simulink model "Citation_FlightGear_v2"  (R2026a)
settings: Solver=ode5  StopTime=10  FixedStep=0.01  EnableMultiTasking=on
InitFcn:
  | run('initcit.m')
  | run('id_init.m')
values from neighbouring files (symbols this model uses):
  beta_ref_max = 5*pi/180    (= 0.0872664625997)    [id_init.m]
  K_beta = 2    [id_init.m]
  K_da_to_p = p_ref_max/0.65    (= 0.537024385229)    [id_init.m]
  K_de_to_q = q_ref_max/0.35    (= 0.49866550057)    [id_init.m]
  K_dr_to_beta = beta_ref_max/0.38    (= 0.229648585789)    [id_init.m]
  Kaw_p = 1/Taw_p    (= 2)    [id_init.m]
  Kaw_q = 1/Taw_q    (= 2)    [id_init.m]
  Kaw_r = 1/Taw_r    (= 2)    [id_init.m]
  Ki_p = 5.0    (= 5)    [id_init.m]
  Ki_p_classical = -0.5    [id_init.m]
  Ki_q = 5.0    (= 5)    [id_init.m]
  Ki_q_classical = -0.1    [id_init.m]
  Ki_r = 5.0    (= 5)    [id_init.m]
  Ki_r_classical = -0.1    [id_init.m]
  Kp_p = 4.5    [id_init.m]
  Kp_p_classical = -1    [id_init.m]
  Kp_q = 4.5    [id_init.m]
  Kp_q_classical = -2    [id_init.m]
  Kp_r = 4.5    [id_init.m]
  Kp_r_classical = -2    [id_init.m]
  p_ref_max = 20*pi/180    (= 0.349065850399)    [id_init.m]
  PL0 = 10000*eye(6)    [id_init.m]
  PM0 = 10000*eye(4)    [id_init.m]
  PN0 = 10000*eye(6)    [id_init.m]
  PX0 = 10000*eye(5)    [id_init.m]
  PY0 = 10000*eye(6)    [id_init.m]
  PZ0 = 10000*eye(4)    [id_init.m]
  q_ref_max = 10*pi/180    (= 0.174532925199)    [id_init.m]
  r_ref_max = 10*pi/180    (= 0.174532925199)    [id_init.m]
  tau_cmd = 0.5    [id_init.m]
  thetaL0 = [       7.0957952465296537e-06 ... (first row only)    [id_init.m]
  thetaM0 = [       1.2280209971618383e-02 ... (first row only)    [id_init.m]
  thetaN0 = [      -4.9609095125384690e-06 ... (first row only)    [id_init.m]
  thetaX0 = zeros(5,1)    [id_init.m]
  thetaY0 = zeros(6,1)    [id_init.m]
  thetaZ0 = zeros(4,1)    [id_init.m]
  TL = 7.0875e-06    [id_init.m]
  TM = 3.2564e-06    [id_init.m]
  TN = 5.4692e-07    [id_init.m]
  TX = 2.2784e-06    [id_init.m]
  TY = 8.0633e-07    [id_init.m]
  TZ = 2.8004e-05    [id_init.m]
  Vw915 = 0    [initcit.m]
  winddir = -27*(pi/180)    (= -0.471238898038)    [initcit.m]
  x0 = []    [cessnac550_3d_sfnc.m]
undefined symbols (not defined in the file or in its folder): chord, cv1, cv2, cv3, cv4, deltagmax1, deltagmax2, deltagmax3, deltagmax4, Deng, ealphag, ealphas, g0, hDME, hGS, kt1, kt2, kt3, lh, massinit, matbuaf, matdaf, matdam, matdbbf, matdeaf, matdgaf, matdqaf, matduaf, matdwaw, matedhr, mateif, matelhr, matemhr, matemv1, matemv2, matemve, matetam, mateuaf, matfaaf, matfaxl, matff, matibaf, matibb, matibmh, matipaf, matipmh, matiraf, matiuaf, matiwaf, matlaf, matlam, matleaf, matleam, matlgaf, matlqaf, matluaf, matmaaf, matmaam, matmaf, matmam ... (+78)
libraries: simulink x13, aerolibfltsims x3, aerolibconvert2 x2, aerolibobsolete x1, aerolibanimutils x1
(part 5 of 5)

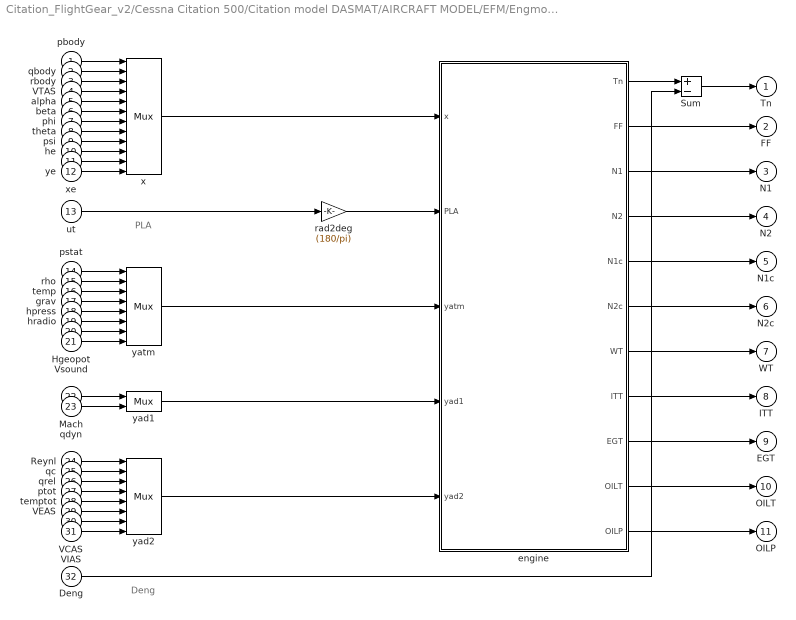
== system Citation_FlightGear_v2/Cessna Citation 500/Citation model DASMAT/AIRCRAFT MODEL/EFM/Engmod/Citation eng_mod/Subsystem1/JT15 Dynamic1/Subsystem ==
  note: Deng
  note: PLA
  pbody : Inport
  qbody : Inport  Port=2
  rbody : Inport  Port=3
  VTAS : Inport  Port=4
  alpha : Inport  Port=5
  beta : Inport  Port=6
  phi : Inport  Port=7
  theta : Inport  Port=8
  psi : Inport  Port=9
  he : Inport  Port=10
  xe : Inport  Port=11
  ye : Inport  Port=12
  ut : Inport  Port=13
  pstat : Inport  Port=14
  rho : Inport  Port=15
  temp : Inport  Port=16
  grav : Inport  Port=17
  hpress : Inport  Port=18
  hradio : Inport  Port=19
  Hgeopot : Inport  Port=20
  Vsound : Inport  Port=21
  Mach : Inport  Port=22
  qdyn : Inport  Port=23
  Reynl : Inport  Port=24
  qc : Inport  Port=25
  qrel : Inport  Port=26
  ptot : Inport  Port=27
  temptot : Inport  Port=28
  VEAS : Inport  Port=29
  VCAS : Inport  Port=30
  VIAS : Inport  Port=31
  Deng : Inport  Port=32
  Sum : Sum  Inputs=+-  InputSameDT=on  SaturateOnIntegerOverflow=on  OutDataTypeStr=Inherit: Same as first input
  engine : Subsystem
  rad2deg : Gain  Gain=(180/pi)  SaturateOnIntegerOverflow=on  OutDataTypeStr=Inherit: Same as input  ParamDataTypeStr=Inherit: Same as input
  x : Mux  Inputs=12
  yad1 : Mux  Inputs=2
  yad2 : Mux  Inputs=8
  yatm : Mux  Inputs=8
  Tn : Outport
  FF : Outport  Port=2
  N1 : Outport  Port=3
  N2 : Outport  Port=4
  N1c : Outport  Port=5
  N2c : Outport  Port=6
  WT : Outport  Port=7
  ITT : Outport  Port=8
  EGT : Outport  Port=9
  OILT : Outport  Port=10
  OILP : Outport  Port=11
  wires:
  Deng/1 -> Sum/2
  engine/1(Tn) -> Sum/1
  Sum/1 -> Tn/1
  Vsound/1 -> yatm/8
  engine/11(OILP) -> OILP/1
  engine/10(OILT) -> OILT/1
  rad2deg/1 -> engine/2(PLA)
  ut/1 -> rad2deg/1
  engine/9(EGT) -> EGT/1
  engine/8(ITT) -> ITT/1
  engine/7(WT) -> WT/1
  engine/6(N2c) -> N2c/1
  engine/5(N1c) -> N1c/1
  engine/4(N2) -> N2/1
  engine/3(N1) -> N1/1
  engine/2(FF) -> FF/1
  yad1/1 -> engine/4(yad1)
  yatm/1 -> engine/3(yatm)
  yad2/1 -> engine/5(yad2)
  qdyn/1 -> yad1/2
  Mach/1 -> yad1/1
  Reynl/1 -> yad2/1
  qc/1 -> yad2/2
  VCAS/1 -> yad2/7
  temptot/1 -> yad2/5
  qrel/1 -> yad2/3
  VIAS/1 -> yad2/8
  VEAS/1 -> yad2/6
  ptot/1 -> yad2/4
  ye/1 -> x/12
  xe/1 -> x/11
  he/1 -> x/10
  psi/1 -> x/9
  VTAS/1 -> x/4
  beta/1 -> x/6
  theta/1 -> x/8
  rbody/1 -> x/3
  alpha/1 -> x/5
  phi/1 -> x/7
  qbody/1 -> x/2
  pbody/1 -> x/1
  pstat/1 -> yatm/1
  rho/1 -> yatm/2
  Hgeopot/1 -> yatm/7
  hpress/1 -> yatm/5
  temp/1 -> yatm/3
  hradio/1 -> yatm/6
  grav/1 -> yatm/4
  x/1 -> engine/1(x)

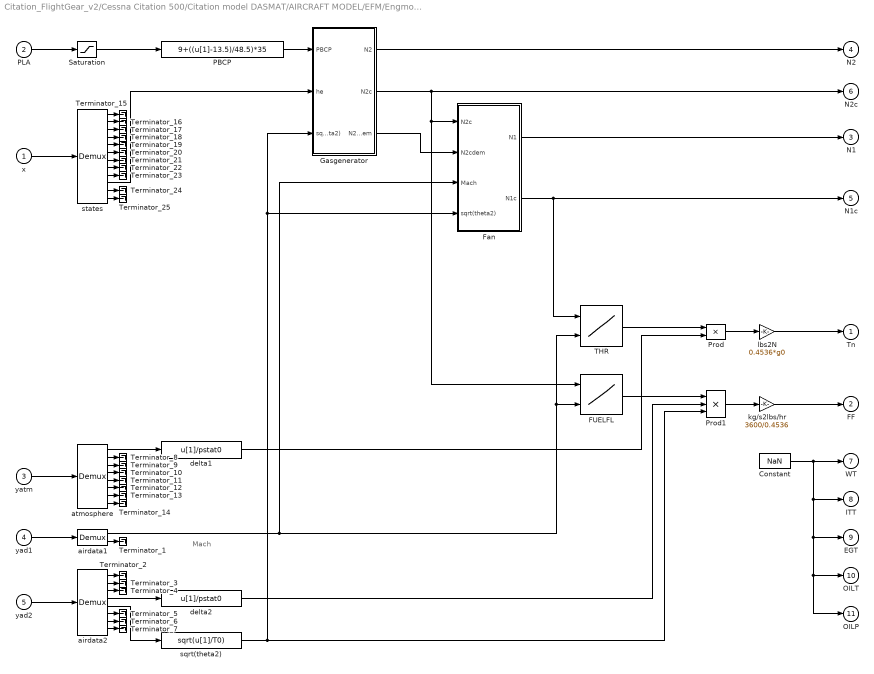
== system Citation_FlightGear_v2/Cessna Citation 500/Citation model DASMAT/AIRCRAFT MODEL/EFM/Engmod/Citation eng_mod/Subsystem1/JT15 Dynamic/Subsystem/engine ==
  note: Mach
  x : Inport
  PLA : Inport  Port=2
  yatm : Inport  Port=3
  yad1 : Inport  Port=4
  yad2 : Inport  Port=5
  Constant : Constant  Value=NaN
  FUELFL : Lookup2D  RowIndex=matff(2:14,1)  ColumnIndex=matff(1,2:14)  Table=matff(2:14,2:14)
  Fan : Subsystem
  Gasgenerator : Subsystem
  PBCP : Fcn  Expr=9+((u[1]-13.5)/48.5)*35
  Prod : Product  InputSameDT=on  SaturateOnIntegerOverflow=on  OutDataTypeStr=Inherit: Same as first input
  Prod1 : Product  Inputs=3  InputSameDT=on  SaturateOnIntegerOverflow=on  OutDataTypeStr=Inherit: Same as first input
  Saturation : Saturate  UpperLimit=62  LowerLimit=13.5
  THR : Lookup2D  RowIndex=matthr(2:12,1)  ColumnIndex=matthr(1,2:12)  Table=matthr(2:12,2:12)
  Terminator_{1..25} (25 alike) : Terminator
  airdata1 : Demux  Outputs=2
      settings: DisplayOption=none
  airdata2 : Demux  Outputs=8
      settings: DisplayOption=none
  atmosphere : Demux  Outputs=8
      settings: DisplayOption=none
  delta1 : Fcn  Expr=u[1]/pstat0
  delta2 : Fcn  Expr=u[1]/pstat0
  kg/s2lbs/hr : Gain  Gain=3600/0.4536  SaturateOnIntegerOverflow=on  OutDataTypeStr=Inherit: Same as input  ParamDataTypeStr=Inherit: Same as input
  lbs2N : Gain  Gain=0.4536*g0  SaturateOnIntegerOverflow=on  OutDataTypeStr=Inherit: Same as input  ParamDataTypeStr=Inherit: Same as input
  sqrt(theta2) : Fcn  Expr=sqrt(u[1]/T0)
  states : Demux  Outputs=12
      settings: DisplayOption=none
  Tn : Outport
  FF : Outport  Port=2
  N1 : Outport  Port=3
  N2 : Outport  Port=4
  N1c : Outport  Port=5
  N2c : Outport  Port=6
  WT : Outport  Port=7
  ITT : Outport  Port=8
  EGT : Outport  Port=9
  OILT : Outport  Port=10
  OILP : Outport  Port=11
  wires:
  states/12 -> Terminator_25/1
  states/11 -> Terminator_24/1
  states/9 -> Terminator_23/1
  states/8 -> Terminator_22/1
  states/7 -> Terminator_21/1
  states/6 -> Terminator_20/1
  states/5 -> Terminator_19/1
  states/4 -> Terminator_18/1
  states/3 -> Terminator_17/1
  states/2 -> Terminator_16/1
  states/1 -> Terminator_15/1
  atmosphere/8 -> Terminator_14/1
  atmosphere/7 -> Terminator_13/1
  atmosphere/6 -> Terminator_12/1
  atmosphere/5 -> Terminator_11/1
  atmosphere/4 -> Terminator_10/1
  atmosphere/3 -> Terminator_9/1
  atmosphere/2 -> Terminator_8/1
  airdata2/8 -> Terminator_7/1
  airdata2/7 -> Terminator_6/1
  airdata2/6 -> Terminator_5/1
  airdata2/3 -> Terminator_4/1
  airdata2/2 -> Terminator_3/1
  airdata2/1 -> Terminator_2/1
  airdata1/2 -> Terminator_1/1
  Fan/2(N1c) -> THR/1, N1c/1
  Gasgenerator/2(N2c) -> Fan/1(N2c), FUELFL/1, N2c/1
  Gasgenerator/3(N2cdem) -> Fan/2(N2cdem)
  airdata1/1 -> Fan/3(Mach), FUELFL/2, THR/2
  Fan/1(N1) -> N1/1
  sqrt(theta2)/1 -> Fan/4(sqrt(theta2)), Gasgenerator/3(sqrt(theta2)), Prod1/3
  yad2/1 -> airdata2/1
  yad1/1 -> airdata1/1
  yatm/1 -> atmosphere/1
  airdata2/4 -> delta2/1
  airdata2/5 -> sqrt(theta2)/1
  Constant/1 -> ITT/1, EGT/1, OILT/1, OILP/1, WT/1
  Gasgenerator/1(N2) -> N2/1
  delta1/1 -> Prod/2
  Prod/1 -> lbs2N/1
  THR/1 -> Prod/1
  lbs2N/1 -> Tn/1
  states/10 -> Gasgenerator/2(he)
  delta2/1 -> Prod1/2
  atmosphere/1 -> delta1/1
  Prod1/1 -> kg/s2lbs/hr/1
  kg/s2lbs/hr/1 -> FF/1
  Saturation/1 -> PBCP/1
  PLA/1 -> Saturation/1
  x/1 -> states/1
  PBCP/1 -> Gasgenerator/1(PBCP)
  FUELFL/1 -> Prod1/1

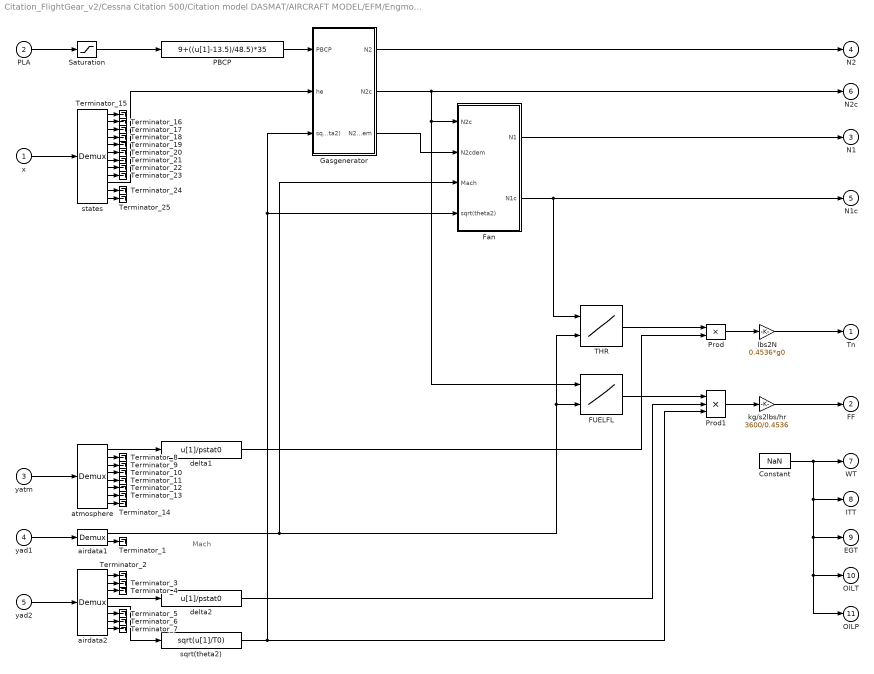
== system Citation_FlightGear_v2/Cessna Citation 500/Citation model DASMAT/AIRCRAFT MODEL/EFM/Engmod/Citation eng_mod/Subsystem1/JT15 Dynamic1/Subsystem/engine ==
  note: Mach
  x : Inport
  PLA : Inport  Port=2
  yatm : Inport  Port=3
  yad1 : Inport  Port=4
  yad2 : Inport  Port=5
  Constant : Constant  Value=NaN
  FUELFL : Lookup2D  RowIndex=matff(2:14,1)  ColumnIndex=matff(1,2:14)  Table=matff(2:14,2:14)
  Fan : Subsystem
  Gasgenerator : Subsystem
  PBCP : Fcn  Expr=9+((u[1]-13.5)/48.5)*35
  Prod : Product  InputSameDT=on  SaturateOnIntegerOverflow=on  OutDataTypeStr=Inherit: Same as first input
  Prod1 : Product  Inputs=3  InputSameDT=on  SaturateOnIntegerOverflow=on  OutDataTypeStr=Inherit: Same as first input
  Saturation : Saturate  UpperLimit=62  LowerLimit=13.5
  THR : Lookup2D  RowIndex=matthr(2:12,1)  ColumnIndex=matthr(1,2:12)  Table=matthr(2:12,2:12)
  Terminator_{1..25} (25 alike) : Terminator
  airdata1 : Demux  Outputs=2
      settings: DisplayOption=none
  airdata2 : Demux  Outputs=8
      settings: DisplayOption=none
  atmosphere : Demux  Outputs=8
      settings: DisplayOption=none
  delta1 : Fcn  Expr=u[1]/pstat0
  delta2 : Fcn  Expr=u[1]/pstat0
  kg/s2lbs/hr : Gain  Gain=3600/0.4536  SaturateOnIntegerOverflow=on  OutDataTypeStr=Inherit: Same as input  ParamDataTypeStr=Inherit: Same as input
  lbs2N : Gain  Gain=0.4536*g0  SaturateOnIntegerOverflow=on  OutDataTypeStr=Inherit: Same as input  ParamDataTypeStr=Inherit: Same as input
  sqrt(theta2) : Fcn  Expr=sqrt(u[1]/T0)
  states : Demux  Outputs=12
      settings: DisplayOption=none
  Tn : Outport
  FF : Outport  Port=2
  N1 : Outport  Port=3
  N2 : Outport  Port=4
  N1c : Outport  Port=5
  N2c : Outport  Port=6
  WT : Outport  Port=7
  ITT : Outport  Port=8
  EGT : Outport  Port=9
  OILT : Outport  Port=10
  OILP : Outport  Port=11
  wires:
  states/12 -> Terminator_25/1
  states/11 -> Terminator_24/1
  states/9 -> Terminator_23/1
  states/8 -> Terminator_22/1
  states/7 -> Terminator_21/1
  states/6 -> Terminator_20/1
  states/5 -> Terminator_19/1
  states/4 -> Terminator_18/1
  states/3 -> Terminator_17/1
  states/2 -> Terminator_16/1
  states/1 -> Terminator_15/1
  atmosphere/8 -> Terminator_14/1
  atmosphere/7 -> Terminator_13/1
  atmosphere/6 -> Terminator_12/1
  atmosphere/5 -> Terminator_11/1
  atmosphere/4 -> Terminator_10/1
  atmosphere/3 -> Terminator_9/1
  atmosphere/2 -> Terminator_8/1
  airdata2/8 -> Terminator_7/1
  airdata2/7 -> Terminator_6/1
  airdata2/6 -> Terminator_5/1
  airdata2/3 -> Terminator_4/1
  airdata2/2 -> Terminator_3/1
  airdata2/1 -> Terminator_2/1
  airdata1/2 -> Terminator_1/1
  Fan/2(N1c) -> THR/1, N1c/1
  Gasgenerator/2(N2c) -> Fan/1(N2c), FUELFL/1, N2c/1
  Gasgenerator/3(N2cdem) -> Fan/2(N2cdem)
  airdata1/1 -> Fan/3(Mach), FUELFL/2, THR/2
  Fan/1(N1) -> N1/1
  sqrt(theta2)/1 -> Fan/4(sqrt(theta2)), Gasgenerator/3(sqrt(theta2)), Prod1/3
  yad2/1 -> airdata2/1
  yad1/1 -> airdata1/1
  yatm/1 -> atmosphere/1
  airdata2/4 -> delta2/1
  airdata2/5 -> sqrt(theta2)/1
  Constant/1 -> ITT/1, EGT/1, OILT/1, OILP/1, WT/1
  Gasgenerator/1(N2) -> N2/1
  delta1/1 -> Prod/2
  Prod/1 -> lbs2N/1
  THR/1 -> Prod/1
  lbs2N/1 -> Tn/1
  states/10 -> Gasgenerator/2(he)
  delta2/1 -> Prod1/2
  atmosphere/1 -> delta1/1
  Prod1/1 -> kg/s2lbs/hr/1
  kg/s2lbs/hr/1 -> FF/1
  Saturation/1 -> PBCP/1
  PLA/1 -> Saturation/1
  x/1 -> states/1
  PBCP/1 -> Gasgenerator/1(PBCP)
  FUELFL/1 -> Prod1/1

== system Citation_FlightGear_v2/Cessna Citation 500/Citation model DASMAT/AIRCRAFT MODEL/EFM/Engmod/Citation eng_mod/Subsystem1/JT15 Dynamic/Subsystem/engine/Fan ==
  note: N1c feedback
  note: N1cdot
  N2c : Inport
  N2cdem : Inport  Port=2
  Mach : Inport  Port=3
  sqrt(theta2) : Inport  Port=4
  Droop : Gain  Gain=2  SaturateOnIntegerOverflow=on  OutDataTypeStr=Inherit: Same as input  ParamDataTypeStr=Inherit: Same as input
  Max accel : Subsystem  mask(Min Value){}
      mask help:
      | Output is minimum value of inputs.
      | y=min(u1,u2)
      mask Help: The Min block produces as output the minimum value of two scalars or vectors. If the inputs are vectors, the output will be a vector containing the minimum elements of the vectors.
      mask Display: disp('Min')
  Max decel : Subsystem  mask(Max Value){}
      mask help:
      | Output is maximum value of inputs.
      | y=max(u1,u2)
      mask Help: The Max block produces as output the maximum value of two scalars or vectors. If the inputs are vectors, the output will be a vector containing the maximum elements of the vectors.
      mask Display: disp('Max')
  N1 state : Integrator  InitialCondition=xt0(2)
  N1D : Lookup2D  RowIndex=matn1d(2:14,1)  ColumnIndex=matn1d(1,2:14)  Table=matn1d(2:14,2:14)
  Prod : Product  InputSameDT=on  SaturateOnIntegerOverflow=on  OutDataTypeStr=Inherit: Same as first input
  Sum : Sum  Inputs=+-  InputSameDT=on  SaturateOnIntegerOverflow=on  OutDataTypeStr=Inherit: Same as first input
  fN1cmax : Lookup  InputValues="[0 25 40 70 94  120]"  Table="[0   0   1   12 14  18]"
  fN1cmin : Lookup  InputValues="[25     50   60   94 100]"  Table="[-0.05  -0.05    -1    -30 -28]"
  N1 : Outport
  N1c : Outport  Port=2
  wires:
  sqrt(theta2)/1 -> Prod/2
  N1 state/1 -> Prod/1, Sum/2, N1c/1
  N2c/1 -> fN1cmin/1, fN1cmax/1
  Max decel/1(out_1) -> N1 state/1
  N1D/1 -> Sum/1
  Max accel/1(out_1) -> Max decel/1(in_1)
  fN1cmax/1 -> Max accel/2(in_2)
  fN1cmin/1 -> Max decel/2(in_2)
  Sum/1 -> Droop/1
  Droop/1 -> Max accel/1(in_1)
  Mach/1 -> N1D/2
  Prod/1 -> N1/1
  N2cdem/1 -> N1D/1

== system Citation_FlightGear_v2/Cessna Citation 500/Citation model DASMAT/AIRCRAFT MODEL/EFM/Engmod/Citation eng_mod/Subsystem1/JT15 Dynamic/Subsystem/engine/Gasgenerator ==
  note: N2 feedback
  note: N2dot
  PBCP : Inport
  he : Inport  Port=2
  sqrt(theta2) : Inport  Port=3
  Droop : Lookup  InputValues=[0 100]  Table="[0.1  2]"
  Fcn : Fcn  Expr=u[1]/u[2]
  Fcn1 : Fcn  Expr=u[1]/u[2]
  Governor : Product  InputSameDT=on  SaturateOnIntegerOverflow=on  OutDataTypeStr=Inherit: Same as first input
  Max accel : Subsystem  mask(Max Value){}
      mask help:
      | Output is maximum value of inputs.
      | y=max(u1,u2)
      mask Help: The Max block produces as output the maximum value of two scalars or vectors. If the inputs are vectors, the output will be a vector containing the maximum elements of the vectors.
      mask Display: disp('Max')
  Min accel : Subsystem  mask(Min Value){}
      mask help:
      | Output is minimum value of inputs.
      | y=min(u1,u2)
      mask Help: The Min block produces as output the minimum value of two scalars or vectors. If the inputs are vectors, the output will be a vector containing the minimum elements of the vectors.
      mask Display: disp('Min')
  Mux : Mux  Inputs=2
  Mux1 : Mux  Inputs=2
  N2 state : Integrator  InitialCondition=xt0(1)
  N2D : Lookup2D  RowIndex=matn2d(2:10,1)  ColumnIndex=matn2d(1,2:10)  Table=matn2d(2:10,2:10)
  Sum : Sum  Inputs=+-  InputSameDT=on  SaturateOnIntegerOverflow=on  OutDataTypeStr=Inherit: Same as first input
  fN2max : Lookup  InputValues=[25 40 70 94]  Table=[0 3 8 10]
  fN2min : Lookup  InputValues="[25     50   60   94 100]"  Table="[-0.05  -0.05    -2    -20 -28]"
  ft2FL : Gain  Gain=.01  SaturateOnIntegerOverflow=on  OutDataTypeStr=Inherit: Same as input  ParamDataTypeStr=Inherit: Same as input
  m2ft : Gain  Gain=(1/0.3048)  SaturateOnIntegerOverflow=on  OutDataTypeStr=Inherit: Same as input  ParamDataTypeStr=Inherit: Same as input
  N2 : Outport
  N2c : Outport  Port=2
  N2cdem : Outport  Port=3
  wires:
  sqrt(theta2)/1 -> Mux1/2, Mux/2
  N2D/1 -> Mux/1, Droop/1, Sum/1
  Fcn1/1 -> N2c/1
  Fcn/1 -> N2cdem/1
  Mux1/1 -> Fcn1/1
  Mux/1 -> Fcn/1
  Min accel/1(out_1) -> Max accel/1(in_1)
  ft2FL/1 -> N2D/2
  m2ft/1 -> ft2FL/1
  he/1 -> m2ft/1
  N2 state/1 -> Mux1/1, fN2min/1, fN2max/1, Sum/2, N2/1
  fN2max/1 -> Min accel/2(in_2)
  fN2min/1 -> Max accel/2(in_2)
  PBCP/1 -> N2D/1
  Droop/1 -> Governor/1
  Sum/1 -> Governor/2
  Governor/1 -> Min accel/1(in_1)
  Max accel/1(out_1) -> N2 state/1

== system Citation_FlightGear_v2/Cessna Citation 500/Citation model DASMAT/AIRCRAFT MODEL/EFM/Engmod/Citation eng_mod/Subsystem1/JT15 Dynamic1/Subsystem/engine/Fan ==
  note: N1c feedback
  note: N1cdot
  N2c : Inport
  N2cdem : Inport  Port=2
  Mach : Inport  Port=3
  sqrt(theta2) : Inport  Port=4
  Droop : Gain  Gain=2  SaturateOnIntegerOverflow=on  OutDataTypeStr=Inherit: Same as input  ParamDataTypeStr=Inherit: Same as input
  Max accel : Subsystem  mask(Min Value){}
      mask help:
      | Output is minimum value of inputs.
      | y=min(u1,u2)
      mask Help: The Min block produces as output the minimum value of two scalars or vectors. If the inputs are vectors, the output will be a vector containing the minimum elements of the vectors.
      mask Display: disp('Min')
  Max decel : Subsystem  mask(Max Value){}
      mask help:
      | Output is maximum value of inputs.
      | y=max(u1,u2)
      mask Help: The Max block produces as output the maximum value of two scalars or vectors. If the inputs are vectors, the output will be a vector containing the maximum elements of the vectors.
      mask Display: disp('Max')
  N1 state : Integrator  InitialCondition=xt0(2)
  N1D : Lookup2D  RowIndex=matn1d(2:14,1)  ColumnIndex=matn1d(1,2:14)  Table=matn1d(2:14,2:14)
  Prod : Product  InputSameDT=on  SaturateOnIntegerOverflow=on  OutDataTypeStr=Inherit: Same as first input
  Sum : Sum  Inputs=+-  InputSameDT=on  SaturateOnIntegerOverflow=on  OutDataTypeStr=Inherit: Same as first input
  fN1cmax : Lookup  InputValues="[0 25 40 70 94  120]"  Table="[0   0   1   12 14  18]"
  fN1cmin : Lookup  InputValues="[25     50   60   94 100]"  Table="[-0.05  -0.05    -1    -30 -28]"
  N1 : Outport
  N1c : Outport  Port=2
  wires:
  sqrt(theta2)/1 -> Prod/2
  N1 state/1 -> Prod/1, Sum/2, N1c/1
  N2c/1 -> fN1cmin/1, fN1cmax/1
  Max decel/1(out_1) -> N1 state/1
  N1D/1 -> Sum/1
  Max accel/1(out_1) -> Max decel/1(in_1)
  fN1cmax/1 -> Max accel/2(in_2)
  fN1cmin/1 -> Max decel/2(in_2)
  Sum/1 -> Droop/1
  Droop/1 -> Max accel/1(in_1)
  Mach/1 -> N1D/2
  Prod/1 -> N1/1
  N2cdem/1 -> N1D/1

== system Citation_FlightGear_v2/Cessna Citation 500/Citation model DASMAT/AIRCRAFT MODEL/EFM/Engmod/Citation eng_mod/Subsystem1/JT15 Dynamic1/Subsystem/engine/Gasgenerator ==
  note: N2 feedback
  note: N2dot
  PBCP : Inport
  he : Inport  Port=2
  sqrt(theta2) : Inport  Port=3
  Droop : Lookup  InputValues=[0 100]  Table="[0.1  2]"
  Fcn : Fcn  Expr=u[1]/u[2]
  Fcn1 : Fcn  Expr=u[1]/u[2]
  Governor : Product  InputSameDT=on  SaturateOnIntegerOverflow=on  OutDataTypeStr=Inherit: Same as first input
  Max accel : Subsystem  mask(Max Value){}
      mask help:
      | Output is maximum value of inputs.
      | y=max(u1,u2)
      mask Help: The Max block produces as output the maximum value of two scalars or vectors. If the inputs are vectors, the output will be a vector containing the maximum elements of the vectors.
      mask Display: disp('Max')
  Min accel : Subsystem  mask(Min Value){}
      mask help:
      | Output is minimum value of inputs.
      | y=min(u1,u2)
      mask Help: The Min block produces as output the minimum value of two scalars or vectors. If the inputs are vectors, the output will be a vector containing the minimum elements of the vectors.
      mask Display: disp('Min')
  Mux : Mux  Inputs=2
  Mux1 : Mux  Inputs=2
  N2 state : Integrator  InitialCondition=xt0(1)
  N2D : Lookup2D  RowIndex=matn2d(2:10,1)  ColumnIndex=matn2d(1,2:10)  Table=matn2d(2:10,2:10)
  Sum : Sum  Inputs=+-  InputSameDT=on  SaturateOnIntegerOverflow=on  OutDataTypeStr=Inherit: Same as first input
  fN2max : Lookup  InputValues=[25 40 70 94]  Table=[0 3 8 10]
  fN2min : Lookup  InputValues="[25     50   60   94 100]"  Table="[-0.05  -0.05    -2    -20 -28]"
  ft2FL : Gain  Gain=.01  SaturateOnIntegerOverflow=on  OutDataTypeStr=Inherit: Same as input  ParamDataTypeStr=Inherit: Same as input
  m2ft : Gain  Gain=(1/0.3048)  SaturateOnIntegerOverflow=on  OutDataTypeStr=Inherit: Same as input  ParamDataTypeStr=Inherit: Same as input
  N2 : Outport
  N2c : Outport  Port=2
  N2cdem : Outport  Port=3
  wires:
  sqrt(theta2)/1 -> Mux1/2, Mux/2
  N2D/1 -> Mux/1, Droop/1, Sum/1
  Fcn1/1 -> N2c/1
  Fcn/1 -> N2cdem/1
  Mux1/1 -> Fcn1/1
  Mux/1 -> Fcn/1
  Min accel/1(out_1) -> Max accel/1(in_1)
  ft2FL/1 -> N2D/2
  m2ft/1 -> ft2FL/1
  he/1 -> m2ft/1
  N2 state/1 -> Mux1/1, fN2min/1, fN2max/1, Sum/2, N2/1
  fN2max/1 -> Min accel/2(in_2)
  fN2min/1 -> Max accel/2(in_2)
  PBCP/1 -> N2D/1
  Droop/1 -> Governor/1
  Sum/1 -> Governor/2
  Governor/1 -> Min accel/1(in_1)
  Max accel/1(out_1) -> N2 state/1

== system Citation_FlightGear_v2/Cessna Citation 500/Citation model DASMAT/AIRCRAFT MODEL/EFM/Engmod/Citation eng_mod/Subsystem1/JT15 Dynamic/Subsystem/engine/Fan/Max accel ==
  in_1 : Inport
  in_2 : Inport  Port=2
  Sum : Sum  Inputs=-+  InputSameDT=on  SaturateOnIntegerOverflow=on  OutDataTypeStr=Inherit: Same as first input
  Switch : Switch
  out_1 : Outport
  wires:
  in_1/1 -> Sum/1, Switch/1
  in_2/1 -> Sum/2, Switch/3
  Sum/1 -> Switch/2
  Switch/1 -> out_1/1

== system Citation_FlightGear_v2/Cessna Citation 500/Citation model DASMAT/AIRCRAFT MODEL/EFM/Engmod/Citation eng_mod/Subsystem1/JT15 Dynamic/Subsystem/engine/Fan/Max decel ==
  in_1 : Inport
  in_2 : Inport  Port=2
  Sum : Sum  Inputs=+-  InputSameDT=on  SaturateOnIntegerOverflow=on  OutDataTypeStr=Inherit: Same as first input
  Switch : Switch
  out_1 : Outport
  wires:
  Switch/1 -> out_1/1
  Sum/1 -> Switch/2
  in_2/1 -> Sum/2, Switch/3
  in_1/1 -> Sum/1, Switch/1

== system Citation_FlightGear_v2/Cessna Citation 500/Citation model DASMAT/AIRCRAFT MODEL/EFM/Engmod/Citation eng_mod/Subsystem1/JT15 Dynamic/Subsystem/engine/Gasgenerator/Max accel ==
  in_1 : Inport
  in_2 : Inport  Port=2
  Sum : Sum  Inputs=+-  InputSameDT=on  SaturateOnIntegerOverflow=on  OutDataTypeStr=Inherit: Same as first input
  Switch : Switch
  out_1 : Outport
  wires:
  Switch/1 -> out_1/1
  Sum/1 -> Switch/2
  in_2/1 -> Sum/2, Switch/3
  in_1/1 -> Sum/1, Switch/1

== system Citation_FlightGear_v2/Cessna Citation 500/Citation model DASMAT/AIRCRAFT MODEL/EFM/Engmod/Citation eng_mod/Subsystem1/JT15 Dynamic/Subsystem/engine/Gasgenerator/Min accel ==
  in_1 : Inport
  in_2 : Inport  Port=2
  Sum : Sum  Inputs=-+  InputSameDT=on  SaturateOnIntegerOverflow=on  OutDataTypeStr=Inherit: Same as first input
  Switch : Switch
  out_1 : Outport
  wires:
  in_1/1 -> Sum/1, Switch/1
  in_2/1 -> Sum/2, Switch/3
  Sum/1 -> Switch/2
  Switch/1 -> out_1/1

== system Citation_FlightGear_v2/Cessna Citation 500/Citation model DASMAT/AIRCRAFT MODEL/EFM/Engmod/Citation eng_mod/Subsystem1/JT15 Dynamic1/Subsystem/engine/Fan/Max accel ==
  in_1 : Inport
  in_2 : Inport  Port=2
  Sum : Sum  Inputs=-+  InputSameDT=on  SaturateOnIntegerOverflow=on  OutDataTypeStr=Inherit: Same as first input
  Switch : Switch
  out_1 : Outport
  wires:
  in_1/1 -> Sum/1, Switch/1
  in_2/1 -> Sum/2, Switch/3
  Sum/1 -> Switch/2
  Switch/1 -> out_1/1

== system Citation_FlightGear_v2/Cessna Citation 500/Citation model DASMAT/AIRCRAFT MODEL/EFM/Engmod/Citation eng_mod/Subsystem1/JT15 Dynamic1/Subsystem/engine/Fan/Max decel ==
  in_1 : Inport
  in_2 : Inport  Port=2
  Sum : Sum  Inputs=+-  InputSameDT=on  SaturateOnIntegerOverflow=on  OutDataTypeStr=Inherit: Same as first input
  Switch : Switch
  out_1 : Outport
  wires:
  Switch/1 -> out_1/1
  Sum/1 -> Switch/2
  in_2/1 -> Sum/2, Switch/3
  in_1/1 -> Sum/1, Switch/1

== system Citation_FlightGear_v2/Cessna Citation 500/Citation model DASMAT/AIRCRAFT MODEL/EFM/Engmod/Citation eng_mod/Subsystem1/JT15 Dynamic1/Subsystem/engine/Gasgenerator/Max accel ==
  in_1 : Inport
  in_2 : Inport  Port=2
  Sum : Sum  Inputs=+-  InputSameDT=on  SaturateOnIntegerOverflow=on  OutDataTypeStr=Inherit: Same as first input
  Switch : Switch
  out_1 : Outport
  wires:
  Switch/1 -> out_1/1
  Sum/1 -> Switch/2
  in_2/1 -> Sum/2, Switch/3
  in_1/1 -> Sum/1, Switch/1

== system Citation_FlightGear_v2/Cessna Citation 500/Citation model DASMAT/AIRCRAFT MODEL/EFM/Engmod/Citation eng_mod/Subsystem1/JT15 Dynamic1/Subsystem/engine/Gasgenerator/Min accel ==
  in_1 : Inport
  in_2 : Inport  Port=2
  Sum : Sum  Inputs=-+  InputSameDT=on  SaturateOnIntegerOverflow=on  OutDataTypeStr=Inherit: Same as first input
  Switch : Switch
  out_1 : Outport
  wires:
  in_1/1 -> Sum/1, Switch/1
  in_2/1 -> Sum/2, Switch/3
  Sum/1 -> Switch/2
  Switch/1 -> out_1/1

== matlab function Citation_FlightGear_v2/RLS for CZ ==
  data: z input; theta_new output; phi input; theta_old input; P_old input; lambda input; reset input; P_new output; yhat output; innovation output
function [theta_new,P_new,yhat,innovation] = ...
    RLS_CZ(z,phi,theta_old,P_old,lambda,reset)

phi = phi(:);

% Previous covariance
Puse = P_old;

% Later used by Step 4
% Reset covariance, not parameter estimate
if reset > 0.5
    n = size(P_old,1);
    Puse = 10000*eye(n);
end

% Prediction using previous parameter estimate
yhat = phi.'*theta_old;

% Innovation
innovation = z - yhat;

% RLS gain
den = lambda + phi.'*Puse*phi;
K = (Puse*phi)/den;

% Parameter update
theta_new = theta_old + K*innovation;

% Covariance update
P_new = (Puse - K*(phi.'*Puse))/lambda;

% Remove numerical asymmetry
P_new = 0.5*(P_new + P_new.');

end

== matlab function Citation_FlightGear_v2/RLS for CL ==
  data: z input; theta_new output; phi input; theta_old input; P_old input; lambda input; reset input; P_new output; yhat output; innovation output
function [theta_new,P_new,yhat,innovation] = ...
    RLS_CL(z,phi,theta_old,P_old,lambda,reset)

phi = phi(:);

% Previous covariance
Puse = P_old;

% Later used by Step 4
% Reset covariance, not parameter estimate
if reset > 0.5
    n = size(P_old,1);
    Puse = 10000*eye(n);
end

% Prediction using previous parameter estimate
yhat = phi.'*theta_old;

% Innovation
innovation = z - yhat;

% RLS gain
den = lambda + phi.'*Puse*phi;
K = (Puse*phi)/den;

% Parameter update
theta_new = theta_old + K*innovation;

% Covariance update
P_new = (Puse - K*(phi.'*Puse))/lambda;

% Remove numerical asymmetry
P_new = 0.5*(P_new + P_new.');

end

== matlab function Citation_FlightGear_v2/RLS for Cm ==
  data: z input; theta_new output; phi input; theta_old input; P_old input; lambda input; reset input; P_new output; yhat output; innovation output
function [theta_new,P_new,yhat,innovation] = ...
    RLS_Cm(z,phi,theta_old,P_old,lambda,reset)

phi = phi(:);

% Previous covariance
Puse = P_old;

% Later used by Step 4
% Reset covariance, not parameter estimate
if reset > 0.5
    n = size(P_old,1);
    Puse = 10000*eye(n);
end

% Prediction using previous parameter estimate
yhat = phi.'*theta_old;

% Innovation
innovation = z - yhat;

% RLS gain
den = lambda + phi.'*Puse*phi;
K = (Puse*phi)/den;

% Parameter update
theta_new = theta_old + K*innovation;

% Covariance update
P_new = (Puse - K*(phi.'*Puse))/lambda;

% Remove numerical asymmetry
P_new = 0.5*(P_new + P_new.');

end

== matlab function Citation_FlightGear_v2/Monitoring Fault Detection/Monitoring Metrics ==
  data: innovations input; MA2 output; AUTOCORR output; VARIANCE output
function [MA2, AUTOCORR, VARIANCE] = monitor_metrics(innovations)
%#codegen

% Number of samples in monitoring window
N = 50;

% Lag used for autocorrelation
kgap = 5;

% Store previous innovation samples
persistent buffer count

if isempty(buffer)
    buffer = zeros(N,6);
    count = 0;
end

% Make sure innovations is a column vector
innovations = innovations(:);

% ---------------------------------------------------------
% Update buffer
% ---------------------------------------------------------

% Move all old values one position backwards
buffer(2:N,:) = buffer(1:N-1,:);

% Put newest innovations at the top
buffer(1,:) = innovations.';

if count < N
    count = count + 1;
end

% Initialize outputs
MA2      = zeros(6,1);
AUTOCORR = zeros(6,1);
VARIANCE = zeros(6,1);

% Do not calculate statistics until buffer is full
if count < N
    return;
end

% ---------------------------------------------------------
% Calculate metrics independently for X,Y,Z,L,M,N
% ---------------------------------------------------------

for j = 1:6

    e = buffer(:,j);

    % 1. Moving average of squared innovation
    MA2(j) = sum(e.^2)/N;

    % 2. Mean innovation
    e_mean = sum(e)/N;

    % 3. Variance
    VARIANCE(j) = sum((e - e_mean).^2)/(N-1);

    % 4. Autocorrelation at lag kgap
    AUTOCORR(j) = ...
        sum(e(1:N-kgap).*e(1+kgap:N))/N;

end

end

== matlab function Citation_FlightGear_v2/CIC lambda_CX ==
  data: z input; lambda_ad output; phi input; theta_old input; P_old input; Sigma0 input; lambda_min input; e output
function [lambda_ad,e] = CIC_lambda( ...
    z,phi,theta_old,P_old,Sigma0,lambda_min)

%#codegen

phi = phi(:);

% Prediction error / innovation
e = z - phi.'*theta_old;

% Information term
s = phi.'*P_old*phi;

% Constant Information Content forgetting factor
lambda_raw = 1 - e^2/(Sigma0*(1 + s));

% Numerical safety
lambda_ad = min(1.0,max(lambda_min,lambda_raw));

end

== matlab function Citation_FlightGear_v2/CIC lambda_CY ==
  data: z input; lambda_ad output; phi input; theta_old input; P_old input; Sigma0 input; lambda_min input; e output
function [lambda_ad,e] = CIC_lambda( ...
    z,phi,theta_old,P_old,Sigma0,lambda_min)

%#codegen

phi = phi(:);

% Prediction error / innovation
e = z - phi.'*theta_old;

% Information term
s = phi.'*P_old*phi;

% Constant Information Content forgetting factor
lambda_raw = 1 - e^2/(Sigma0*(1 + s));

% Numerical safety
lambda_ad = min(1.0,max(lambda_min,lambda_raw));

end

== matlab function Citation_FlightGear_v2/CIC lambda_CZ ==
  data: z input; lambda_ad output; phi input; theta_old input; P_old input; Sigma0 input; lambda_min input; e output
function [lambda_ad,e] = CIC_lambda( ...
    z,phi,theta_old,P_old,Sigma0,lambda_min)

%#codegen

phi = phi(:);

% Prediction error / innovation
e = z - phi.'*theta_old;

% Information term
s = phi.'*P_old*phi;

% Constant Information Content forgetting factor
lambda_raw = 1 - e^2/(Sigma0*(1 + s));

% Numerical safety
lambda_ad = min(1.0,max(lambda_min,lambda_raw));

end

== matlab function Citation_FlightGear_v2/CIC lambda_Cl ==
  data: z input; lambda_ad output; phi input; theta_old input; P_old input; Sigma0 input; lambda_min input; e output
function [lambda_ad,e] = CIC_lambda( ...
    z,phi,theta_old,P_old,Sigma0,lambda_min)

%#codegen

phi = phi(:);

% Prediction error / innovation
e = z - phi.'*theta_old;

% Information term
s = phi.'*P_old*phi;

% Constant Information Content forgetting factor
lambda_raw = 1 - e^2/(Sigma0*(1 + s));

% Numerical safety
lambda_ad = min(1.0,max(lambda_min,lambda_raw));

end

== matlab function Citation_FlightGear_v2/CIC lambda_Cm ==
  data: z input; lambda_ad output; phi input; theta_old input; P_old input; Sigma0 input; lambda_min input; e output
function [lambda_ad,e] = CIC_lambda( ...
    z,phi,theta_old,P_old,Sigma0,lambda_min)

%#codegen

phi = phi(:);

% Prediction error / innovation
e = z - phi.'*theta_old;

% Information term
s = phi.'*P_old*phi;

% Constant Information Content forgetting factor
lambda_raw = 1 - e^2/(Sigma0*(1 + s));

% Numerical safety
lambda_ad = min(1.0,max(lambda_min,lambda_raw));

end

== matlab function Citation_FlightGear_v2/CIC lambda_Cn ==
  data: z input; lambda_ad output; phi input; theta_old input; P_old input; Sigma0 input; lambda_min input; e output
function [lambda_ad,e] = CIC_lambda( ...
    z,phi,theta_old,P_old,Sigma0,lambda_min)

%#codegen

phi = phi(:);

% Prediction error / innovation
e = z - phi.'*theta_old;

% Information term
s = phi.'*P_old*phi;

% Constant Information Content forgetting factor
lambda_raw = 1 - e^2/(Sigma0*(1 + s));

% Numerical safety
lambda_ad = min(1.0,max(lambda_min,lambda_raw));

end

== matlab function Citation_FlightGear_v2/ANDI Rate Controller/ANDI Inversion ==
  data: nu input; u_model output; p input; q input; r input; V input; alpha input; beta input; rho input; thetaL input; thetaM input; thetaN input; valid_B output; nu_aw output; u_unsat_model output; sat_vec output
function [u_model,valid_B,nu_aw,u_unsat_model,sat_vec] = ...
    ANDI_Inversion(nu,p,q,r,V,alpha,beta,rho,thetaL,thetaM,thetaN)

% ==========================================================
% Default outputs
% Ensures every output is assigned on every execution path
% ==========================================================
u_model       = zeros(3,1);
u_unsat_model = zeros(3,1);
nu_aw         = zeros(3,1);
sat_vec       = false(3,1);

valid_B = false;

u_ndi_unsat = zeros(3,1);
u_ndi_sat   = zeros(3,1);

u_model = zeros(3,1);
valid_B = false;

u_ndi = zeros(3,1);

% ==========================================================
% Aircraft constants
% ==========================================================

Ixx = 11187.8;
Iyy = 22854.8;
Izz = 31974.8;
Ixz = 1930.1;

S = 24.9900;
b = 13.3250;
c = 1.9910;

I = [ Ixx,  0,   -Ixz;
       0,   Iyy,   0;
     -Ixz,  0,    Izz];

omega = [p;q;r];

% ==========================================================
% Identified Cl derivatives
%
% thetaL =
% [Cl0 Clbeta Clp Clr Clda Cldr]'
% ==========================================================

Cl0    = thetaL(1);
Clbeta = thetaL(2);
Clp    = thetaL(3);
Clr    = thetaL(4);
Clda   = thetaL(5);
Cldr   = thetaL(6);

% ==========================================================
% Identified Cm derivatives
%
% thetaM =
% [Cm0 Cmalpha Cmq Cmde]'
% ==========================================================

Cm0     = thetaM(1);
Cmalpha = thetaM(2);
Cmq     = thetaM(3);
Cmde    = thetaM(4);

% ==========================================================
% Identified Cn derivatives
%
% thetaN =
% [Cn0 Cnbeta Cnp Cnr Cnda Cndr]'
% ==========================================================

Cn0    = thetaN(1);
Cnbeta = thetaN(2);
Cnp    = thetaN(3);
Cnr    = thetaN(4);
Cnda   = thetaN(5);
Cndr   = thetaN(6);

% ==========================================================
% Protect against division by zero
% ==========================================================

if V < 1
    return
end

% ==========================================================
% Dimensionless angular rates
% Must match the RLS regressors exactly
% ==========================================================

phat = p*b/(2*V);
qhat = q*c/V;
rhat = r*b/(2*V);

% ==========================================================
% Aerodynamic moment coefficients excluding controls
% ==========================================================

Cl_free = Cl0 ...
        + Clbeta*beta ...
        + Clp*phat ...
        + Clr*rhat;

Cm_free = Cm0 ...
        + Cmalpha*alpha ...
        + Cmq*qhat;

Cn_free = Cn0 ...
        + Cnbeta*beta ...
        + Cnp*phat ...
        + Cnr*rhat;

% ==========================================================
% Dynamic pressure
% ==========================================================

qbar = 0.5*rho*V^2;

% ==========================================================
% State-dependent aerodynamic moment vector
% ==========================================================

M0 = qbar*S * ...
    [b*Cl_free;
     c*Cm_free;
     b*Cn_free];

% ==========================================================
% Control-effectiveness matrix
%
% NDI input order:
%
%       [da de dr]'
% ==========================================================

G = qbar*S * ...
    [b*Clda,   0,       b*Cldr;
     0,        c*Cmde,  0;
     b*Cnda,   0,       b*Cndr];

% ==========================================================
% Nonlinear gyroscopic term
% ==========================================================

gyro = cross(omega,I*omega);

% ==========================================================
% Rotational model
%
% omega_dot = a(x) + B(x)u
% ==========================================================

a = I \ (M0 - gyro);

B = I \ G;

% ==========================================================
% Check whether B is sufficiently invertible
% ==========================================================

if rcond(B) > 1e-6

    % Requested surface commands
    % NDI order = [da de dr]'
    u_ndi_unsat = B \ (nu-a);

    % ------------------------------------------------------
    % Surface saturation
    % ------------------------------------------------------

    da_sat = min(max(u_ndi_unsat(1), -0.65),  0.65);
    de_sat = min(max(u_ndi_unsat(2), -0.35),  0.26);
    dr_sat = min(max(u_ndi_unsat(3), -0.38),  0.38);

    u_ndi_sat = [da_sat;
                 de_sat;
                 dr_sat];

    % ------------------------------------------------------
    % Anti-windup discrepancy
    % ------------------------------------------------------

    delta_u = u_ndi_sat - u_ndi_unsat;

    % Convert actuator saturation back into virtual-control
    % coordinates.
    nu_aw = B * delta_u;

    % Useful for logging / diagnostics
    sat_vec = abs(delta_u) > 1e-8;

    valid_B = true;

end

% Requested unsaturated Citation-order command
u_unsat_model = [u_ndi_unsat(2);
                 u_ndi_unsat(1);
                 u_ndi_unsat(3)];

% Command actually sent toward Citation actuator model
u_model = [u_ndi_sat(2);
           u_ndi_sat(1);
           u_ndi_sat(3)];

end

== matlab function Citation_FlightGear_v2/Regressors Symmetr. and Asymmetr. F//M Coefficients ==
  data: alpha input; beta input; p input; q input; r input; V input; de input; da input; dr input; phiX output; phiZM output; phiLat output
function [phiX,phiZM,phiLat] = ...
    build_regressors(alpha,beta,p,q,r,V,de,da,dr)

% Aircraft geometry
b = 13.3250;
c = 1.9910;

% Dimensionless angular-rate terms
qhat = q*c/V;
phat = p*b/(2*V);
rhat = r*b/(2*V);

% CX
phiX = [1;
        alpha;
        alpha^2;
        qhat;
        de];

% CZ and Cm
phiZM = [1;
         alpha;
         qhat;
         de];

% CY, Cl and Cn
phiLat = [1;
          beta;
          phat;
          rhat;
          da;
          dr];

end

== matlab function Citation_FlightGear_v2/Calculation of Force//Moments Coefficients ==
  data: p input; CX output; q input; r input; pdot input; qdot input; rdot input; V input; h input; anxb input; anyb input; anzb input; CY output; CZ output; Cl output; Cm output; Cn output; rho output
function [CX,CY,CZ,Cl,Cm,Cn,rho] = ...
    aero_measurements(p,q,r,pdot,qdot,rdot,V,h,anxb,anyb,anzb)

% Aircraft constants
m   = 4500;

Ixx = 11187.8;
Iyy = 22854.8;
Izz = 31974.8;
Ixz = 1930.1;

S = 24.9900;
b = 13.3250;
c = 1.9910;

% Atmosphere
g0     = 9.80665;
R      = 287.05;
lambda = -0.0065;
T0     = 288.15;
rho0   = 1.225;
htrop  = 11000;

% Density
Ttrop = T0 + lambda*htrop;

rho_trop = rho0 * (1 + lambda*htrop/T0)^(-g0/(R*lambda)-1);

if h <= htrop
    rho = rho0 * (1 + lambda*h/T0)^(-g0/(R*lambda)-1);
else
    rho = rho_trop * exp(-g0*(h-htrop)/(R*Ttrop));
end

% Convert specific forces from g to m/s^2
Ax = anxb*g0;
Ay = anyb*g0;
Az = anzb*g0;

% Dynamic pressure
qbar = 0.5*rho*V^2;

% Force coefficients
CX = m*Ax/(qbar*S);
CY = m*Ay/(qbar*S);
CZ = m*Az/(qbar*S);

% Aerodynamic moments from rigid-body rotational equations
L = Ixx*pdot + q*r*(Izz-Iyy) - (p*q + rdot)*Ixz;

M = Iyy*qdot + r*p*(Ixx-Izz) + (p^2-r^2)*Ixz;

N = Izz*rdot + p*q*(Iyy-Ixx) + (q*r-pdot)*Ixz;

% Moment coefficients
Cl = L/(qbar*S*b);
Cm = M/(qbar*S*c);
Cn = N/(qbar*S*b);

end

== matlab function Citation_FlightGear_v2/RLS for Cn ==
  data: z input; theta_new output; phi input; theta_old input; P_old input; lambda input; reset input; P_new output; yhat output; innovation output
function [theta_new,P_new,yhat,innovation] = ...
    RLS_Cn(z,phi,theta_old,P_old,lambda,reset)

phi = phi(:);

% Previous covariance
Puse = P_old;

% Later used by Step 4
% Reset covariance, not parameter estimate
if reset > 0.5
    n = size(P_old,1);
    Puse = 10000*eye(n);
end

% Prediction using previous parameter estimate
yhat = phi.'*theta_old;

% Innovation
innovation = z - yhat;

% RLS gain
den = lambda + phi.'*Puse*phi;
K = (Puse*phi)/den;

% Parameter update
theta_new = theta_old + K*innovation;

% Covariance update
P_new = (Puse - K*(phi.'*Puse))/lambda;

% Remove numerical asymmetry
P_new = 0.5*(P_new + P_new.');

end

== matlab function Citation_FlightGear_v2/RLS for CX ==
  data: z input; theta_new output; phi input; theta_old input; P_old input; lambda input; reset input; P_new output; yhat output; innovation output
function [theta_new,P_new,yhat,innovation] = ...
    RLS_CX(z,phi,theta_old,P_old,lambda,reset)

phi = phi(:);

% Previous covariance
Puse = P_old;

% Later used by Step 4
% Reset covariance, not parameter estimate
if reset > 0.5
    n = size(P_old,1);
    Puse = 10000*eye(n);
end

% Prediction using previous parameter estimate
yhat = phi.'*theta_old;

% Innovation
innovation = z - yhat;

% RLS gain
den = lambda + phi.'*Puse*phi;
K = (Puse*phi)/den;

% Parameter update
theta_new = theta_old + K*innovation;

% Covariance update
P_new = (Puse - K*(phi.'*Puse))/lambda;

% Remove numerical asymmetry
P_new = 0.5*(P_new + P_new.');

end

== matlab function Citation_FlightGear_v2/RLS for CY ==
  data: z input; theta_new output; phi input; theta_old input; P_old input; lambda input; reset input; P_new output; yhat output; innovation output
function [theta_new,P_new,yhat,innovation] = ...
    RLS_CY(z,phi,theta_old,P_old,lambda,reset)

phi = phi(:);

% Previous covariance
Puse = P_old;

% Later used by Step 4
% Reset covariance, not parameter estimate
if reset > 0.5
    n = size(P_old,1);
    Puse = 10000*eye(n);
end

% Prediction using previous parameter estimate
yhat = phi.'*theta_old;

% Innovation
innovation = z - yhat;

% RLS gain
den = lambda + phi.'*Puse*phi;
K = (Puse*phi)/den;

% Parameter update
theta_new = theta_old + K*innovation;

% Covariance update
P_new = (Puse - K*(phi.'*Puse))/lambda;

% Remove numerical asymmetry
P_new = 0.5*(P_new + P_new.');

end
